simulink model "sim_1_1"  (R2021b)
settings: Solver=ode4  StartTime=0.0  StopTime=tstop  FixedStep=tstep  RelTol=1e-3
values from neighbouring files (symbols this model uses):
  C = 0.01    [sim_1.m]
  L = 0.1    [sim_1.m]
  R = 99    [sim_1.m]
settings Model: Creator=shash  LastModifiedBy=shash
settings DataIOCC: ReturnWorkspaceOutputs=off

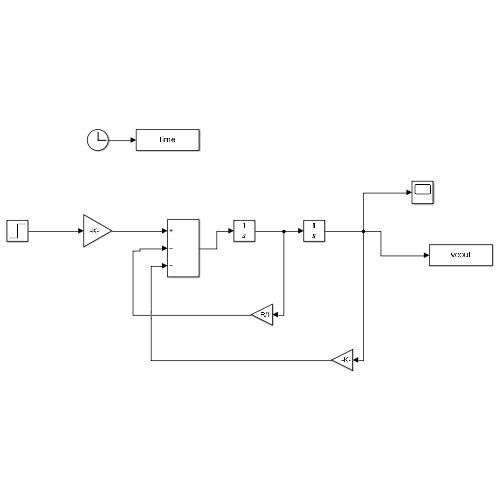
[thumbnail: Simulink's stored preview of the top-level diagram]
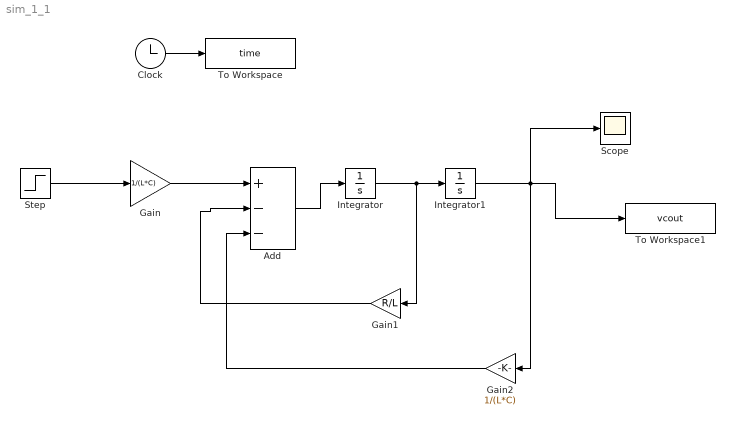
== system sim_1_1 ==
  Add : Sum  Inputs=+--
  Clock : Clock
  Gain : Gain  Gain=1/(L*C)
  Gain1 : Gain  Gain=R/L
  Gain2 : Gain  Gain=1/(L*C)
  Integrator : Integrator
  Integrator1 : Integrator
  Scope : Scope
  Step : Step  Time=0  SampleTime=0
  To Workspace : ToWorkspace  VariableName=time  SampleTime=-1
  To Workspace1 : ToWorkspace  VariableName=vcout  SampleTime=-1
  wires:
  Gain/1 -> Add/1
  Add/1 -> Integrator/1
  Integrator/1 -> Gain1/1, Integrator1/1
  Gain1/1 -> Add/2
  Gain2/1 -> Add/3
  Step/1 -> Gain/1
  Integrator1/1 -> Scope/1, Gain2/1, To Workspace1/1
  Clock/1 -> To Workspace/1
